simulink model "TDM"  (R2017b)
settings: Solver=VariableStepAuto  StartTime=0.0  StopTime=10  RelTol=1e-3
libraries: dsparch4 x1, simulink x1
settings Model: Creator=ayadd  LastModifiedBy=ayadd

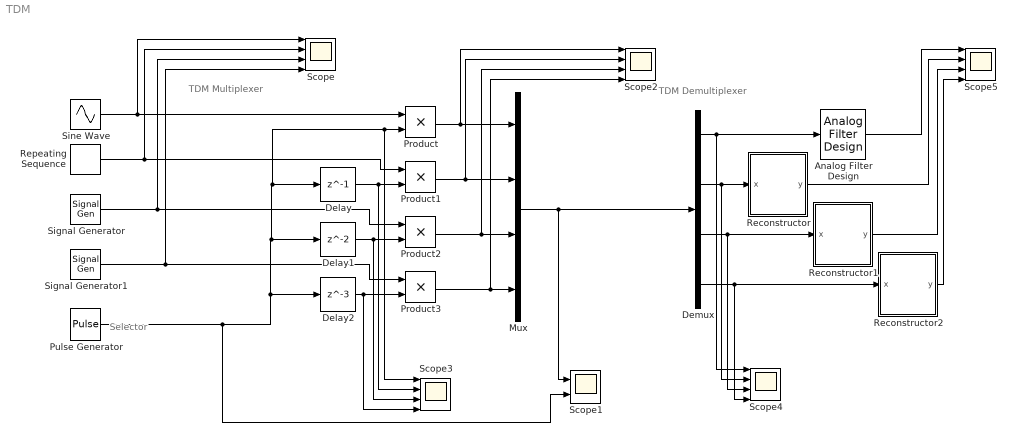
== system TDM ==
  note: TDM Demultiplexer
  note: Selector
  note: TDM Multiplexer
  Analog Filter Design : dsparch4/Analog Filter Design  method=Butterworth  filttype=Lowpass  N=8  Wlo=10*2*pi  Whi=80  Rp=2  Rs=40
  Delay : Delay  DelayLength=1  InitialCondition=0  SampleTime=0.00025
  Delay1 : Delay  SampleTime=0.00025
  Delay2 : Delay  DelayLength=3  SampleTime=0.00025
  Demux : Demux
  Mux : Mux
  Product{,1..3} (4 alike) : Product
  Pulse Generator : DiscretePulseGenerator  PulseType=Time based  Period=0.001  PulseWidth=25
  Reconstructor : Subsystem
  Reconstructor1 : Subsystem
  Reconstructor2 : Subsystem
  Repeating Sequence : simulink/Sources/Repeating Sequence  rep_seq_t=[0 0.5]  rep_seq_y=[0 2]
  Scope{,2..5} (5 alike) : Scope  NumInputPorts=4
  Scope1 : Scope  NumInputPorts=2
  Signal Generator : SignalGenerator  WaveForm=sawtooth  Frequency=10
  Signal Generator1 : SignalGenerator  WaveForm=square  Frequency=10
  Sine Wave : Sin  Frequency=4*2*pi  SampleTime=0
  wires:
  Mux/1 -> Demux/1, Scope1/1
  Sine Wave/1 -> Scope/1, Product/1
  Product1/1 -> Scope2/2, Mux/2
  Delay/1 -> Scope3/2, Product1/2
  Product/1 -> Scope2/1, Mux/1
  Product2/1 -> Scope2/3, Mux/3
  Repeating Sequence/1 -> Scope/2, Product1/1
  Signal Generator1/1 -> Scope/4, Product3/1
  Signal Generator/1 -> Scope/3, Product2/1
  Product3/1 -> Scope2/4, Mux/4
  Delay2/1 -> Scope3/4, Product3/2
  Delay1/1 -> Scope3/3, Product2/2
  Pulse Generator/1 -> Scope1/2, Product/2, Scope3/1, Delay/1, Delay1/1, Delay2/1
  Demux/1 -> Analog Filter Design/1, Scope4/1
  Demux/3 -> Reconstructor1/1(x), Scope4/3
  Demux/4 -> Reconstructor2/1(x), Scope4/4
  Analog Filter Design/1 -> Scope5/1
  Reconstructor2/1(y) -> Scope5/4
  Demux/2 -> Reconstructor/1(x), Scope4/2
  Reconstructor/1(y) -> Scope5/2
  Reconstructor1/1(y) -> Scope5/3

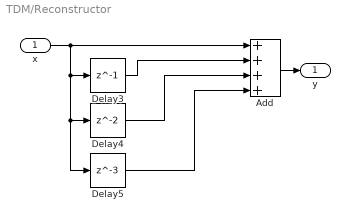
== system TDM/Reconstructor ==
  x : Inport
  Add : Sum  Inputs=++++
  Delay3 : Delay  DelayLength=1  InitialCondition=0  SampleTime=0.00025
  Delay4 : Delay  InitialCondition=0  SampleTime=0.00025
  Delay5 : Delay  DelayLength=3  InitialCondition=0  SampleTime=0.00025
  y : Outport
  wires:
  Delay3/1 -> Add/2
  Delay4/1 -> Add/3
  Delay5/1 -> Add/4
  Add/1 -> y/1
  x/1 -> Delay5/1, Delay4/1, Delay3/1, Add/1

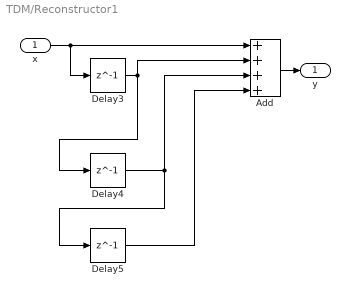
== system TDM/Reconstructor1 ==
  x : Inport
  Add : Sum  Inputs=++++
  Delay3 : Delay  DelayLength=1  InitialCondition=0  SampleTime=0.00025
  Delay4 : Delay  DelayLength=1  InitialCondition=0  SampleTime=0.00025
  Delay5 : Delay  DelayLength=1  InitialCondition=0  SampleTime=0.00025
  y : Outport
  wires:
  Delay3/1 -> Delay4/1, Add/2
  Delay4/1 -> Add/3, Delay5/1
  Delay5/1 -> Add/4
  Add/1 -> y/1
  x/1 -> Delay3/1, Add/1

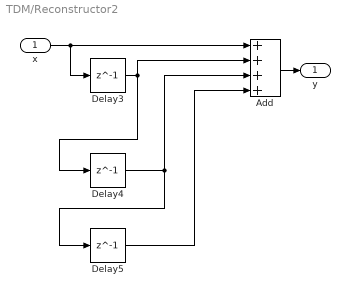
== system TDM/Reconstructor2 ==
  x : Inport
  Add : Sum  Inputs=++++
  Delay3 : Delay  DelayLength=1  InitialCondition=0  SampleTime=0.00025
  Delay4 : Delay  DelayLength=1  InitialCondition=0  SampleTime=0.00025
  Delay5 : Delay  DelayLength=1  InitialCondition=0  SampleTime=0.00025
  y : Outport
  wires:
  Delay3/1 -> Delay4/1, Add/2
  Delay4/1 -> Add/3, Delay5/1
  Delay5/1 -> Add/4
  Add/1 -> y/1
  x/1 -> Delay3/1, Add/1
